simulink model "rx_byte_aligner_32bit"  (R2024a)
settings: Solver=FixedStepDiscrete  StartTime=0.0  StopTime=1  RelTol=1e-3
settings Model: Creator=User  LastModifiedBy=Vetaly
settings SolverCC: AlgebraicLoopSolver=TrustRegion
settings DataIOCC: LimitDataPoints=on  SaveFormat=Array  SignalLoggingSaveFormat=ModelDataLogs  SaveOutput=off  SignalLogging=off  SaveTime=off  ReturnWorkspaceOutputs=off
settings OptimizationCC: BlockReduction=off  ConditionallyExecuteInputs=off  DefaultParameterBehavior=Inlined  ExpressionDepthLimit=2147483647  LifeSpan=inf
settings DebuggingCC: AlgebraicLoopMsg=error  ArtificialAlgebraicLoopMsg=none  UnderspecifiedInitializationDetection=Classic  MergeDetectMultiDrivingBlocksExec=none  InheritedTsInSrcMsg=none  SingleTaskRateTransMsg=error  IntegerOverflowMsg=none  FcnCallInpInsideContextMsg=warning  ModelReferenceSymbolNameMessage=none  StateNameClashWarn=warning  SFUnexpectedBacktrackingDiag=warning  SFNoUnconditionalDefaultTransitionDiag=warning  SFExecutionAtInitializationDiag=none  IntegerSaturationMsg=none  ArithmeticOperatorsInVariantConditions=warning
settings HardwareCC: ProdBitPerPointer=32  ProdBitPerSizeT=32  ProdBitPerPtrDiffT=32  ProdLargestAtomicFloat=None  ProdIntDivRoundTo=Undefined  ProdEndianess=Unspecified  ProdWordSize=32  ProdHWDeviceType=ASIC/FPGA->ASIC/FPGA  ProdEqTarget=off
settings ModelReferenceCC: EnableRefExpFcnMdlSchedulingChecks=on  ModelReferenceMinAlgLoopOccurrences=on  PropagateSignalLabelsOutOfModel=off
settings SFSimCC: SimUseLocalCustomCode=off  SimParseCustomCode=off  CustomCodeUndefinedFunction=UseInterfaceOnly
settings RTWCC: RTWVerbose=off  RTWUseLocalCustomCode=off  RTWCompilerOptimization=on  GPUComputeCapability=3.5  DLArmComputeVersion=19.05
settings CodeAppCC: StateflowObjectComments=on
settings GRTTargetCC: TargetLangStandard=C89/C90 (ANSI)  CombineOutputUpdateFcns=off  GRTInterface=on
settings ConfigComp: CovMetricSettings=dw  CovSaveCumulativeToWorkspaceVar=on  CovSaveSingleToWorkspaceVar=on  CovExternalEMLEnable=off

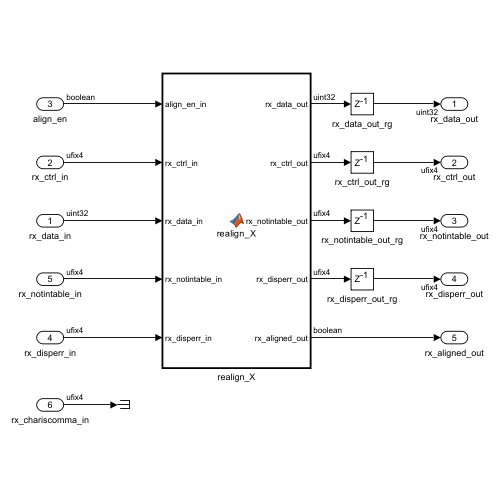
[thumbnail: Simulink's stored preview of the top-level diagram]
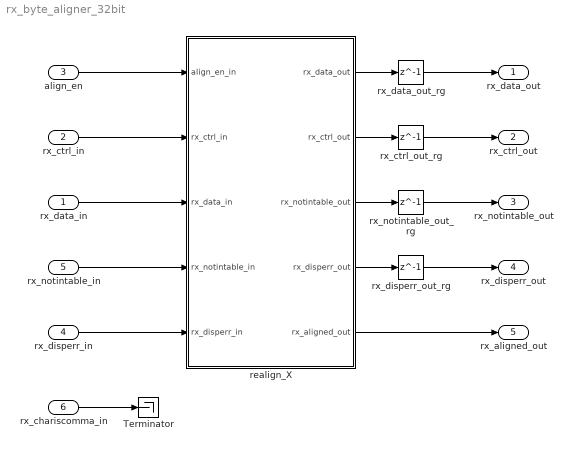
== system rx_byte_aligner_32bit ==
  rx_data_in : Inport  OutDataTypeStr=uint32
  rx_ctrl_in : Inport  Port=2  OutDataTypeStr=fixdt(0,4,0)
  align_en : Inport  Port=3  OutDataTypeStr=boolean
  rx_disperr_in : Inport  Port=4  OutDataTypeStr=fixdt(0,4,0)
  rx_notintable_in : Inport  Port=5  OutDataTypeStr=fixdt(0,4,0)
  rx_chariscomma_in : Inport  Port=6  OutDataTypeStr=fixdt(0,4,0)
  Terminator : Terminator
  realign_X : MATLAB Function  TreatAsAtomicUnit=on
  rx_ctrl_out_rg : Delay  DelayLength=1
  rx_data_out_rg : Delay  DelayLength=1
  rx_disperr_out_rg : Delay  DelayLength=1
  rx_notintable_out_rg : Delay  DelayLength=1
  rx_data_out : Outport
  rx_ctrl_out : Outport  Port=2
  rx_notintable_out : Outport  Port=3
  rx_disperr_out : Outport  Port=4
  rx_aligned_out : Outport  Port=5
  wires:
  rx_data_in/1 -> realign_X/3(rx_data_in)
  rx_ctrl_in/1 -> realign_X/2(rx_ctrl_in)
  realign_X/1(rx_data_out) -> rx_data_out_rg/1
  rx_notintable_in/1 -> realign_X/4(rx_notintable_in)
  rx_disperr_in/1 -> realign_X/5(rx_disperr_in)
  rx_chariscomma_in/1 -> Terminator/1
  realign_X/2(rx_ctrl_out) -> rx_ctrl_out_rg/1
  realign_X/3(rx_notintable_out) -> rx_notintable_out_rg/1
  realign_X/4(rx_disperr_out) -> rx_disperr_out_rg/1
  realign_X/5(rx_aligned_out) -> rx_aligned_out/1
  align_en/1 -> realign_X/1(align_en_in)
  rx_data_out_rg/1 -> rx_data_out/1
  rx_ctrl_out_rg/1 -> rx_ctrl_out/1
  rx_notintable_out_rg/1 -> rx_notintable_out/1
  rx_disperr_out_rg/1 -> rx_disperr_out/1

== matlab function rx_byte_aligner_32bit/realign_X ==
  settings: sampleTime=1
  settings: fimath=|
      | fimath(...
      | 'RoundMode', 'floor',...
      | 'OverflowMode', 'wrap',...
      | 'ProductMode', 'FullPrecision', 'ProductWordLength', 16,...
      | 'SumMode', 'FullPrecision', 'SumWordLength', 16,...
      | 'CastBeforeSum', true)
  data: align_en_in input; rx_data_out output; rx_ctrl_out output; rx_ctrl_in input; rx_data_in input; rx_notintable_in input; rx_notintable_out output; rx_disperr_in input; rx_disperr_out output; rx_aligned_out output
function [rx_data_out, rx_ctrl_out, rx_notintable_out,rx_disperr_out, rx_aligned_out] = realign_X(align_en_in, rx_ctrl_in, rx_data_in, rx_notintable_in, rx_disperr_in)
fm = fimath('OverflowMode','Wrap');

COMMA_BYTE = 0xBC;

persistent rx_data_d rx_ctrl_d rx_err_d rx_disperr_d have_prev rx_aligned
% persistent first_ALIGNp_received_r;
persistent shift_r;

if isempty(rx_data_d)
    have_prev = false;
    rx_data_d = uint32(0);
    rx_ctrl_d = fi(0,0,4,0,fm);
    rx_err_d = fi(0,0,4,0,fm);
    rx_disperr_d = fi(0,0,4,0,fm);
    % first_ALIGNp_received_r = false;
    shift_r = fi(0,0,2,0,fm);
    rx_aligned = false;
end

rx_aligned_out = rx_aligned;
% rx_aligned_out = first_ALIGNp_received_r;


%% -------- байты текущего (сырого) слова --------
b0 = bitsliceget(fi(rx_data_in,0,32,0,fm),8,1); % rx_data[7:0];
b1 = bitsliceget(fi(rx_data_in,0,32,0,fm),16,9); % rx_data[15:8];
b2 = bitsliceget(fi(rx_data_in,0,32,0,fm),24,17); % rx_data[23:16];
b3 = bitsliceget(fi(rx_data_in,0,32,0,fm),32,25); % rx_data[31:24];

comma0 = bitget(rx_ctrl_in,1)==1 && b0==COMMA_BYTE;
comma1 = bitget(rx_ctrl_in,2)==1 && b1==COMMA_BYTE;
comma2 = bitget(rx_ctrl_in,3)==1 && b2==COMMA_BYTE;
comma3 = bitget(rx_ctrl_in,4)==1 && b3==COMMA_BYTE;

%% -------- one-hot декодер: и позиция, и валидность одним case'ом --------
switch uint8(bitconcat(fi(comma3,0,1,0,fm), fi(comma2,0,1,0,fm), fi(comma1,0,1,0,fm), fi(comma0,0,1,0,fm)))
    case bin2dec('0001')
        comma_ok = true;s_detect = fi(0,0,shift_r.WordLength,0,fm);
    case bin2dec('0010')
        comma_ok = true;s_detect = fi(3,0,shift_r.WordLength,0,fm);
    case bin2dec('0100')
        comma_ok = true;s_detect = fi(2,0,shift_r.WordLength,0,fm);
    case bin2dec('1000')
        comma_ok = true;s_detect = fi(1,0,shift_r.WordLength,0,fm);
    otherwise
        comma_ok = false;s_detect = fi(0,0,shift_r.WordLength,0,fm); % 0000 или >1 бита - игнор
end

% align_en = ~first_ALIGNp_received_r;
align_en = align_en_in;

update_shift = align_en && comma_ok;
% shift_now = update_shift ? s_detect : shift_r;
if (update_shift)
    shift_now = fi(s_detect, 0, shift_r.WordLength, 0, fm);
else
    shift_now = fi(shift_r, 0, shift_r.WordLength, 0, fm);
end

% фиксация сдвига:
if (update_shift)
    shift_r = s_detect;
end

if (update_shift && have_prev)
    rx_aligned = true;
end


switch shift_now
    case 0
        rx_data_out = uint32(rx_data_in);
        rx_ctrl_out = fi(rx_ctrl_in,0,4,0,fm);
        rx_notintable_out = fi(rx_notintable_in,0,4,0,fm);
        rx_disperr_out = fi(rx_disperr_in,0,4,0,fm);

    case 1
        rx_data_out = uint32( bitconcat( bitsliceget(fi(rx_data_in,0,32,0,fm),24,1), bitsliceget(fi(rx_data_d,0,32,0,fm),32,25)) );
        rx_ctrl_out = bitconcat( bitsliceget(rx_ctrl_in,3,1), bitget(rx_ctrl_d,4));
        rx_notintable_out = bitconcat( bitsliceget(rx_notintable_in,3,1), bitget(rx_err_d,4));
        rx_disperr_out = bitconcat( bitsliceget(rx_disperr_in,3,1), bitget(rx_disperr_d,4));

    case 2
        rx_data_out = uint32( bitconcat( bitsliceget(fi(rx_data_in,0,32,0,fm),16,1), bitsliceget(fi(rx_data_d,0,32,0,fm),32,17)) );
        rx_ctrl_out = bitconcat( bitsliceget(rx_ctrl_in,2,1), bitsliceget(rx_ctrl_d,4,3));
        rx_notintable_out = bitconcat( bitsliceget(rx_notintable_in,2,1), bitsliceget(rx_err_d,4,3));
        rx_disperr_out = bitconcat( bitsliceget(rx_disperr_in,2,1), bitsliceget(rx_disperr_d,4,3));

    otherwise
        rx_data_out = uint32( bitconcat( bitsliceget(fi(rx_data_in,0,32,0,fm),8,1), bitsliceget(fi(rx_data_d,0,32,0,fm),32,9)) );
        rx_ctrl_out = bitconcat( bitget(rx_ctrl_in,1), bitsliceget(rx_ctrl_d,4,2));
        rx_notintable_out = bitconcat( bitget(rx_notintable_in,1), bitsliceget(rx_err_d,4,2));
        rx_disperr_out = bitconcat( bitget(rx_disperr_in,1), bitsliceget(rx_disperr_d,4,2));
end

% if (~PHYRDY)
%     first_ALIGNp_received_r = false;
%     % have_prev = false;
% else
%     % if (rx_data_out==hex2dec('7B4A4ABC') && rx_ctrl_out==1)
%     if (rx_data_out==hex2dec('7B4A4ABC') && rx_ctrl_out==1 && rx_notintable_out==0)
%         first_ALIGNp_received_r = true;
%     end
% end



rx_data_d = uint32(rx_data_in);
rx_ctrl_d = fi(rx_ctrl_in,0,4,0,fm);
rx_err_d = fi(rx_notintable_in,0,4,0,fm);
rx_disperr_d = fi(rx_disperr_in,0,4,0,fm);
have_prev = true;
